simulink library "NullTcasSurveillanceBus"  (R2018b)
settings: Solver=VariableStepAuto  StartTime=0.0  StopTime=10.0  RelTol=1e-3
settings Model: Creator=RA24876  LastModifiedBy=RA24876
settings SFSimCC: SimUseLocalCustomCode=off
settings RTWCC: RTWUseLocalCustomCode=off
settings CodeAppCC: StateflowObjectComments=on

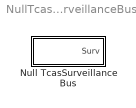
== system NullTcasSurveillanceBus ==
  Null TcasSurveillance Bus : Subsystem  mask(Null TcasSurveillance Bus){}
      mask help: Creates a TcasSurveillance bus signal with all null values. Assign values to elements with a Bus Assignment block.

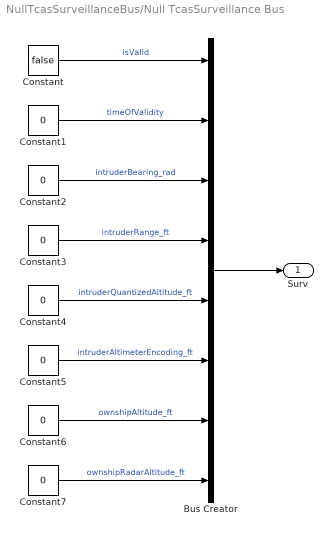
== system NullTcasSurveillanceBus/Null TcasSurveillance Bus ==
  Bus Creator : BusCreator  Inputs=8  OutDataTypeStr=Bus: TcasSurveillance
      settings: InheritFromInputs=off
  Constant : Constant  Value=false  OutDataTypeStr=boolean
  Constant{1..7} (7 alike) : Constant  Value=0
  Surv : Outport  OutDataTypeStr=Bus: TcasSurveillance
  wires:
  Constant6/1 -> Bus Creator/7  "ownshipAltitude_ft"
  Constant7/1 -> Bus Creator/8  "ownshipRadarAltitude_ft"
  Constant2/1 -> Bus Creator/3  "intruderBearing_rad"
  Constant/1 -> Bus Creator/1  "isValid"
  Constant3/1 -> Bus Creator/4  "intruderRange_ft"
  Constant5/1 -> Bus Creator/6  "intruderAltimeterEncoding_ft"
  Constant4/1 -> Bus Creator/5  "intruderQuantizedAltitude_ft"
  Bus Creator/1 -> Surv/1
  Constant1/1 -> Bus Creator/2  "timeOfValidity"
